simulink model "exercise_01_simscape"  (R2022b)
settings: Solver=VariableStepAuto  StartTime=0.0  StopTime=10*2*pi/w  MaxStep=(2*pi/w)*1e-4  MinStep=(2*pi/w)*1e-12  RelTol=1e-3  AbsTol=1e-3
model workspace (MAT data in the model file):
  C = 0.5
  L = 2
  R = 1
  alpha = -1
  w = 6.28318530718
libraries: fl_lib x12, nesl_utility x5
settings Model: Creator=paolo  LastModifiedBy=stefa
settings SolverCC: AutoScaleAbsTol=off  AlgebraicLoopSolver=TrustRegion  MaxZcPerStep=1
settings DebuggingCC: UnconnectedInputMsg=warning  UnconnectedOutputMsg=warning  UnconnectedLineMsg=warning  SymbolicDimsDataTypeCodeGenerationDiagnostic=none
settings ModelReferenceCC: EnableRefExpFcnMdlSchedulingChecks=on
settings SFSimCC: CustomCodeUndefinedFunction=UseInterfaceOnly
settings RTWCC: DLArmComputeVersion=19.05
settings SimscapeCC: SimscapeLogType=all  SimscapeLogSimulationStatistics=on  SimscapeLogDataHistory=10000

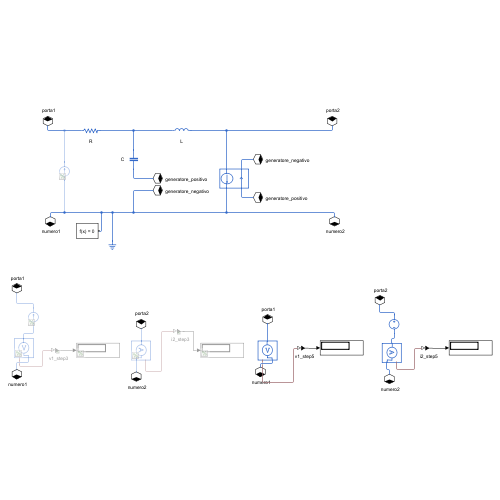
[thumbnail: Simulink's stored preview of the top-level diagram]
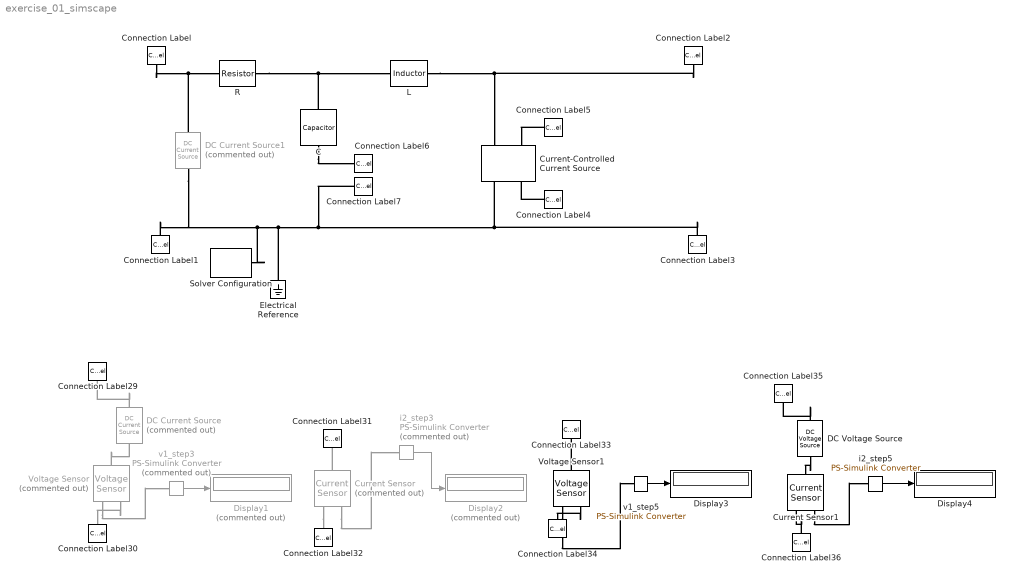
== system exercise_01_simscape ==
  C : fl_lib/Electrical/Electrical Elements/Capacitor  c=C F  r=0 Ohm  g=0 1/Ohm  i_specify=off  i_priority=None  i=0 A  i_nominal_specify=off  i_nominal_unit=A  i_nominal_value=1  v_specify=off  v_priority=None  v=0 V  v_nominal_specify=off  v_nominal_unit=V  v_nominal_value=1  vc_specify=off  vc_priority=High  vc=0 V  vc_nominal_specify=off  vc_nominal_unit=V  vc_nominal_value=1
  Connection Label : ConnectionLabel  Label=porta1
  Connection Label1 : ConnectionLabel  Label=numero1
  Connection Label2 : ConnectionLabel  Label=porta2
  Connection Label29 : ConnectionLabel  Label=porta1
  Connection Label3 : ConnectionLabel  Label=numero2
  Connection Label30 : ConnectionLabel  Label=numero1
  Connection Label31 : ConnectionLabel  Label=porta2
  Connection Label32 : ConnectionLabel  Label=numero2
  Connection Label33 : ConnectionLabel  Label=porta1
  Connection Label34 : ConnectionLabel  Label=numero1
  Connection Label35 : ConnectionLabel  Label=porta2
  Connection Label36 : ConnectionLabel  Label=numero2
  Connection Label4 : ConnectionLabel  Label=generatore_positivo
  Connection Label5 : ConnectionLabel  Label=generatore_negativo
  Connection Label6 : ConnectionLabel  Label=generatore_positivo
  Connection Label7 : ConnectionLabel  Label=generatore_negativo
  Current Sensor : fl_lib/Electrical/Electrical Sensors/Current Sensor  Commented=on
  Current Sensor1 : fl_lib/Electrical/Electrical Sensors/Current Sensor
  Current-Controlled Current Source : fl_lib/Electrical/Electrical Sources/Current-Controlled Current Source  K=alpha  i1_specify=off  i1_priority=None  i1=0 A  i1_nominal_specify=off  i1_nominal_unit=A  i1_nominal_value=1  i2_specify=off  i2_priority=None  i2=0 A  i2_nominal_specify=off  i2_nominal_unit=A  i2_nominal_value=1
      settings: InternalSimscapePortConfiguration="{\"Bottom\":[],\"Left\":[{\"id\":\"p1\",\"label\":\"+\",\"type\":\"foundation.electrical.electrical\"},{\"id\":\"head\",\"label\":\"\",\"type\":\"foundation.electrical.electrical\"}],\"Right\":[{\"id\":\"n1\",\"label\":\"-\",\"type\":\"foundation.electrical.electrical\"},{\"id\":\"tail\",\"label\":\"\",\"type\":\"foundation.electrical.electrical\"}],\"Top\":[]}"
  DC Current Source : fl_lib/Electrical/Electrical Sources/DC Current Source  Commented=on  i0=1 A
      settings: InternalSimscapePortConfiguration="{\"Bottom\":[],\"Left\":[{\"id\":\"p\",\"label\":\"\",\"type\":\"foundation.electrical.electrical\"}],\"Right\":[{\"id\":\"n\",\"label\":\"\",\"type\":\"foundation.electrical.electrical\"}],\"Top\":[]}"
  DC Current Source1 : fl_lib/Electrical/Electrical Sources/DC Current Source  Commented=on  i0=1 A
      settings: InternalSimscapePortConfiguration="{\"Bottom\":[],\"Left\":[{\"id\":\"p\",\"label\":\"\",\"type\":\"foundation.electrical.electrical\"}],\"Right\":[{\"id\":\"n\",\"label\":\"\",\"type\":\"foundation.electrical.electrical\"}],\"Top\":[]}"
  DC Voltage Source : fl_lib/Electrical/Electrical Sources/DC Voltage Source  v0=1 V
  Display1 : Display  Commented=on
  Display2 : Display  Commented=on
  Display3 : Display
  Display4 : Display
  Electrical Reference : fl_lib/Electrical/Electrical Elements/Electrical Reference
  L : fl_lib/Electrical/Electrical Elements/Inductor  l=L H  r=0 Ohm  g=0 1/Ohm  i_specify=off  i_priority=None  i=0 A  i_nominal_specify=off  i_nominal_unit=A  i_nominal_value=1  v_specify=off  v_priority=None  v=0 V  v_nominal_specify=off  v_nominal_unit=V  v_nominal_value=1  i_L_specify=off  i_L_priority=High  i_L=0 A  i_L_nominal_specify=off  i_L_nominal_unit=A  i_L_nominal_value=1
  R : fl_lib/Electrical/Electrical Elements/Resistor  R=R Ohm  i_specify=off  i_priority=None  i=0 A  i_nominal_specify=off  i_nominal_unit=A  i_nominal_value=1  v_specify=off  v_priority=None  v=0 V  v_nominal_specify=off  v_nominal_unit=V  v_nominal_value=1
  Solver Configuration : nesl_utility/Solver Configuration  PhysicalDomain=network_engine_domain  SubClassName=solver  LeftPortType=input  RightPortType=generic  Tones=[]  Harmonics=[]  SimulateNoise=off  Profile=off  UseLocalSampling=off  EnableSwitchedLinearOptims=on  FrequencyDomain=off  UseCCode=off  RelTol=0.001  AbsTol=0.001  MinStep=1e-09  ToWorkspace=off  RevertToSquareIcSolve=off  NumHomotopyIterations=100  PhasorMode=off  PhasorModeNumHarmonics=1  ConsistencySolver=NEWTON_XTOL_AFTER_FTOL  IndexReductionMethod=DerivativeReplacement  DoDC=off  ResidualTolerance=1e-09  ConsistencyTolSource=GLOBAL  ConsistencyAbsTol=0.001  ConsistencyRelTol=0.001  ConsistencyTolFactor=0.001  UseLocalSolver=off  LocalSolverChoice=NE_BACKWARD_EULER_ADVANCER  ResolveIndetEquations=on  FunctionEvalNumThread=1  LocalSolverSampleTime=0.001  DoFixedCost=off  MaxNonlinIter=3  MaxModeIter=2  ComputeImpulses=off  ImpulseIterations=2  LinearAlgebra=auto  LinearAlgebraNumThread=0  EquationFormulation=NE_TIME_EF  DelaysMemoryBudget=1024  AutomaticFiltering=on  FilteringTimeConstant=0.001  PartitionStorageMethod=AS_NEEDED  PartitionMemoryBudget=1024  PartitionMethod=ROBUST
  Voltage Sensor : fl_lib/Electrical/Electrical Sensors/Voltage Sensor  Commented=on
  Voltage Sensor1 : fl_lib/Electrical/Electrical Sensors/Voltage Sensor
  i2_step3 : nesl_utility/PS-Simulink Converter  Commented=on  PhysicalDomain=network_engine_domain  SubClassName=ps_output  LeftPortType=input  RightPortType=output  PseudoPeriodic=off  Frequencies=[]  VectorFormat=1-D array  Unit=inherit  AffineConversion=off
  i2_step5 : nesl_utility/PS-Simulink Converter  PhysicalDomain=network_engine_domain  SubClassName=ps_output  LeftPortType=input  RightPortType=output  PseudoPeriodic=off  Frequencies=[]  VectorFormat=1-D array  Unit=inherit  AffineConversion=off
  v1_step3 : nesl_utility/PS-Simulink Converter  Commented=on  PhysicalDomain=network_engine_domain  SubClassName=ps_output  LeftPortType=input  RightPortType=output  PseudoPeriodic=off  Frequencies=[]  VectorFormat=1-D array  Unit=inherit  AffineConversion=off
  v1_step5 : nesl_utility/PS-Simulink Converter  PhysicalDomain=network_engine_domain  SubClassName=ps_output  LeftPortType=input  RightPortType=output  PseudoPeriodic=off  Frequencies=[]  VectorFormat=1-D array  Unit=inherit  AffineConversion=off
  wires:
  i2_step3/1 -> Display2/1
  v1_step5/1 -> Display3/1
  i2_step5/1 -> Display4/1
  v1_step3/1 -> Display1/1
  connections:
  R/RConn1 -- C/LConn1 -- L/LConn1
  DC Current Source1/RConn1 -- Connection Label1/LConn1 -- Solver Configuration/RConn1 -- Electrical Reference/LConn1 -- Connection Label7/LConn1 -- Connection Label3/LConn1 -- Current-Controlled Current Source/LConn2
  Connection Label/LConn1 -- DC Current Source1/LConn1 -- R/LConn1
  Connection Label5/LConn1 -- Current-Controlled Current Source/RConn1
  Connection Label4/LConn1 -- Current-Controlled Current Source/LConn1
  Connection Label2/LConn1 -- L/RConn1 -- Current-Controlled Current Source/RConn2
  Current Sensor1/RConn1 -- i2_step5/LConn1
  Connection Label36/LConn1 -- Current Sensor1/RConn2
  Voltage Sensor1/RConn1 -- v1_step5/LConn1
  DC Voltage Source/RConn1 -- Current Sensor1/LConn1
  Current Sensor/RConn1 -- i2_step3/LConn1
  Voltage Sensor/RConn2 -- Connection Label30/LConn1
  Voltage Sensor1/LConn1 -- Connection Label33/LConn1
  Voltage Sensor1/RConn2 -- Connection Label34/LConn1
  Current Sensor/RConn2 -- Connection Label32/LConn1
  Current Sensor/LConn1 -- Connection Label31/LConn1
  Voltage Sensor/RConn1 -- v1_step3/LConn1
  Voltage Sensor/LConn1 -- DC Current Source/RConn1
  DC Voltage Source/LConn1 -- Connection Label35/LConn1
  DC Current Source/LConn1 -- Connection Label29/LConn1
  C/RConn1 -- Connection Label6/LConn1
